simulink model "model_4"  (R2020b)
settings: Solver=VariableStepAuto  StartTime=0.0  StopTime=10.0  RelTol=1e-3
settings Model: Creator=Chetan  LastModifiedBy=Chetan

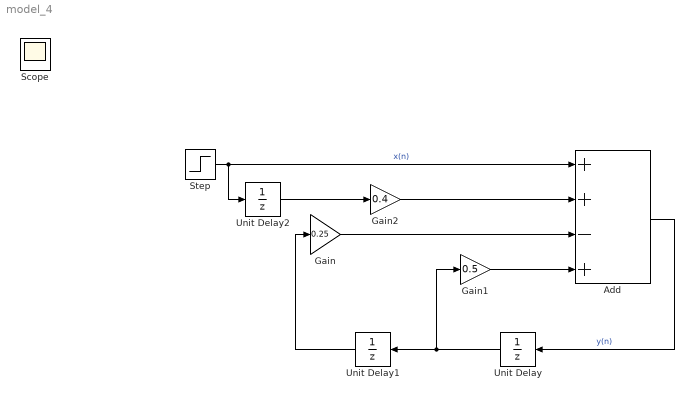
== system model_4 ==
  Add : Sum  Inputs=++-+
  Gain : Gain  Gain=0.25
  Gain1 : Gain  Gain=0.5
  Gain2 : Gain  Gain=0.4
  Step : Step  SampleTime=0
  Unit Delay : UnitDelay  SampleTime=-1  HasFrameUpgradeWarning=on
  Unit Delay1 : UnitDelay  SampleTime=-1  HasFrameUpgradeWarning=on
  Unit Delay2 : UnitDelay  SampleTime=-1  HasFrameUpgradeWarning=on
  Scope : Scope
  wires:
  Unit Delay/1 -> Gain1/1, Unit Delay1/1
  Add/1 -> Unit Delay/1  "y(n)"
  Gain/1 -> Add/3
  Unit Delay1/1 -> Gain/1
  Gain1/1 -> Add/4
  Step/1 -> Unit Delay2/1, Add/1  "x(n)"
  Gain2/1 -> Add/2
  Unit Delay2/1 -> Gain2/1
